simulink model "Sposob_1b"  (R2022b)
settings: Solver=ode4  StartTime=0.0  StopTime=10.0  FixedStep=0.1  RelTol=1e-3
values from neighbouring files (symbols this model uses):
  F = 1    [Sposob1.mat]    (also in Sposob2a.mat; Sposob2b.mat; Sposob3a.mat; Sposob3b.mat)
  k = 6    [Sposob1.mat]    (also in Sposob2a.mat; Sposob2b.mat; Sposob3a.mat; Sposob3b.mat)
  m = 14    [Sposob1.mat]    (also in Sposob2a.mat; Sposob2b.mat; Sposob3a.mat; Sposob3b.mat)
  x0 = 0.1    [Sposob1.mat]    (also in Sposob2a.mat = [0.1 0]; Sposob2b.mat = [0.1 0]; Sposob3a.mat = [0.1 0]; Sposob3b.mat = [0.1 0])
settings Model: Creator=student  LastModifiedBy=Jakub
settings DebuggingCC: UnconnectedInputMsg=warning  UnconnectedOutputMsg=warning  UnconnectedLineMsg=warning
settings ModelReferenceCC: EnableRefExpFcnMdlSchedulingChecks=on
settings RTWCC: DLArmComputeVersion=19.05

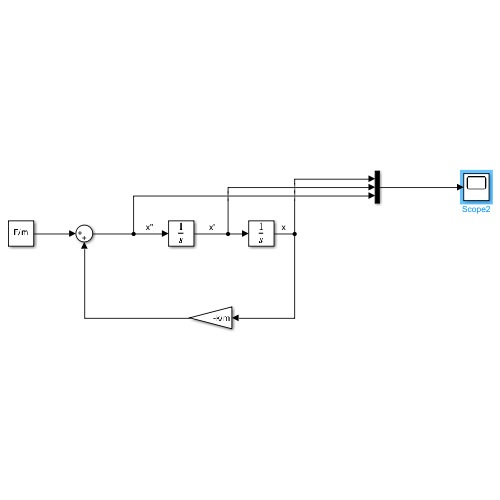
[thumbnail: Simulink's stored preview of the top-level diagram]
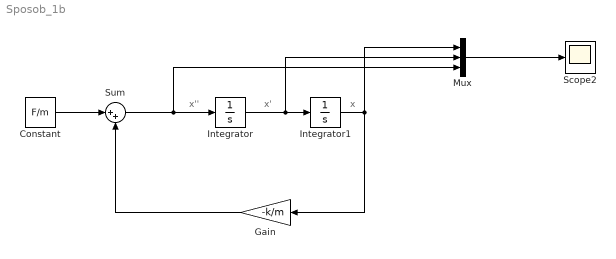
== system Sposob_1b ==
  note: x
  note: x'
  note: x''
  Constant : Constant  Value=F/m
  Gain : Gain  Gain=-k/m
  Integrator : Integrator
  Integrator1 : Integrator  InitialCondition=x0
  Mux : Mux  Inputs=3
  Scope2 : Scope
  Sum : Sum  Inputs=|++
  wires:
  Integrator/1 -> Mux/2, Integrator1/1
  Integrator1/1 -> Mux/1, Gain/1
  Mux/1 -> Scope2/1
  Constant/1 -> Sum/1
  Gain/1 -> Sum/2
  Sum/1 -> Mux/3, Integrator/1
